simulink subsystem "Clase_Leds"  (R2023b)
settings: Solver=VariableStepAuto  StartTime=0.0  StopTime=10.0  RelTol=1e-3
libraries: arduinolib x3, simulink x1
settings Model: Creator=Andrés  LastModifiedBy=Andrés

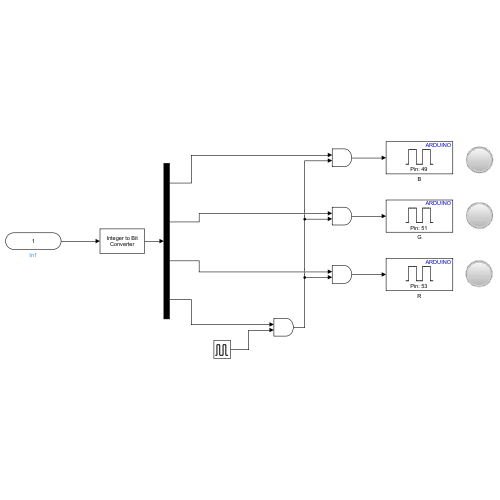
[thumbnail: Simulink's stored preview of the top-level diagram]
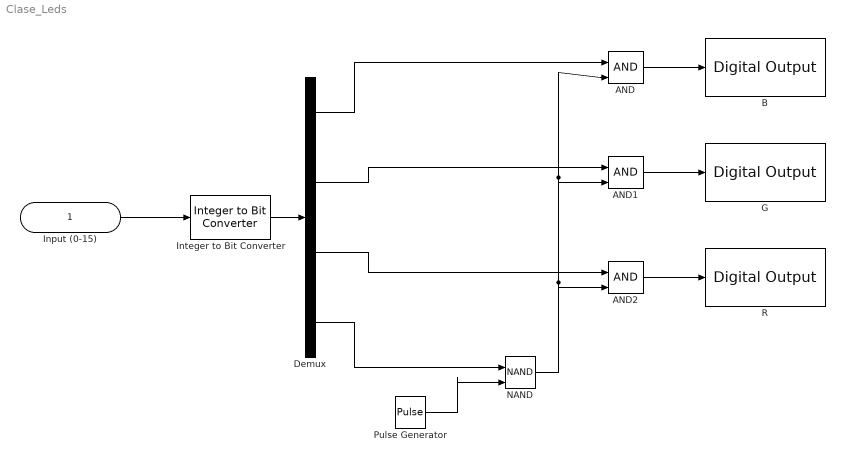
== system Clase_Leds ==
  Input (0-15) : Inport
  AND : Logic  IconShape=distinctive  AllPortsSameDT=off  OutDataTypeStr=boolean
  AND1 : Logic  IconShape=distinctive  AllPortsSameDT=off  OutDataTypeStr=boolean
  AND2 : Logic  IconShape=distinctive  AllPortsSameDT=off  OutDataTypeStr=boolean
  B : arduinolib/Digital Output  pinNumber=49  Direction=output  blockPlatform=arduino
  Demux : Demux
  G : arduinolib/Digital Output  pinNumber=51  Direction=output  blockPlatform=arduino
  Integer to Bit Converter : simulink/Logic and Bit Operations/Integer to Bit Converter  nbits=4  signedInputValues=Unsigned  bitOrder=MSB first  outDtype=Inherit via internal rule
  NAND : Logic  Operator=NAND  IconShape=distinctive  AllPortsSameDT=off  OutDataTypeStr=boolean
  Pulse Generator : DiscretePulseGenerator  PulseType=Time based  PulseWidth=50
  R : arduinolib/Digital Output  pinNumber=53  Direction=output  blockPlatform=arduino
  wires:
  AND1/1 -> G/1
  AND/1 -> B/1
  AND2/1 -> R/1
  Input (0-15)/1 -> Integer to Bit Converter/1
  Integer to Bit Converter/1 -> Demux/1
  NAND/1 -> AND/2, AND1/2, AND2/2
  Pulse Generator/1 -> NAND/2
  Demux/4 -> NAND/1
  Demux/3 -> AND2/1
  Demux/2 -> AND1/1
  Demux/1 -> AND/1
